simulink model "PIDDiscreto"  (R2021a)
settings: Solver=VariableStepAuto  StartTime=0.0  StopTime=60  RelTol=1e-3
values from neighbouring files (symbols this model uses):
  g = 9.81    [Parcial2PIDDiscreto.m]
  L = 0.25    [Parcial2PIDDiscreto.m]
  m = 0.03    [Parcial2PIDDiscreto.m]
  M = 0.510    (= 0.51)    [Parcial2PIDDiscreto.m]
  ts = 5    [Parcial2PIDDiscreto.m]
  Ts = 0.1    [Parcial2PIDDiscreto.m]
undefined symbols (not defined in the file or in its folder): kdc, kdp, kic, kip, kpc, kpp, Nc, Np
libraries: spsStairGeneratorLib x1
settings Model: Creator=manue  LastModifiedBy=manue

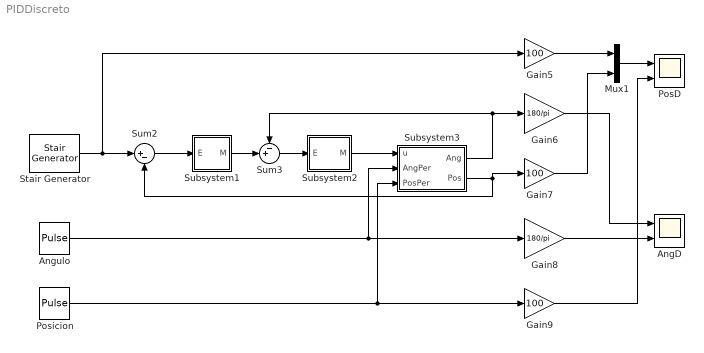
== system PIDDiscreto ==
  AngD : Scope  NumInputPorts=2
  Angulo : DiscretePulseGenerator  PulseType=Time based  Amplitude=10*pi/180  Period=60  PulseWidth=0.1  PhaseDelay=20
  Gain5 : Gain  Gain=100
  Gain6 : Gain  Gain=180/pi
  Gain7 : Gain  Gain=100
  Gain8 : Gain  Gain=180/pi
  Gain9 : Gain  Gain=100
  Mux1 : Mux  Inputs=2
  PosD : Scope  NumInputPorts=2
  Posicion : DiscretePulseGenerator  PulseType=Time based  Amplitude=5/100  Period=60  PhaseDelay=40
  Stair Generator : spsStairGeneratorLib/Stair Generator  t=[0, ts,2*ts,3*ts,4*ts,5*ts,6*ts,7*ts,8*ts,9*ts,10*ts]  e=[25,35,35,40,40,35,35,10,10,30,30]/100  Ts=0
  Subsystem1 : Subsystem
  Subsystem2 : Subsystem
  Subsystem3 : Subsystem
  Sum2 : Sum  Inputs=|+-
  Sum3 : Sum  Inputs=-+|
  wires:
  Gain9/1 -> PosD/2
  Gain5/1 -> Mux1/1
  Posicion/1 -> Subsystem3/3(PosPer), Gain9/1
  Angulo/1 -> Subsystem3/2(AngPer), Gain8/1
  Subsystem3/2(Pos) -> Gain7/1, Sum2/2
  Stair Generator/1 -> Gain5/1, Sum2/1
  Gain6/1 -> AngD/1
  Gain8/1 -> AngD/2
  Subsystem3/1(Ang) -> Sum3/1, Gain6/1
  Gain7/1 -> Mux1/2
  Mux1/1 -> PosD/1
  Sum3/1 -> Subsystem2/1(E)
  Sum2/1 -> Subsystem1/1(E)
  Subsystem1/1(M) -> Sum3/2
  Subsystem2/1(M) -> Subsystem3/1(u)

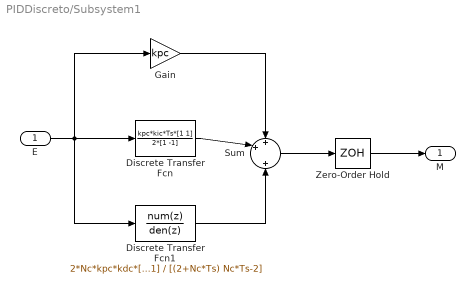
== system PIDDiscreto/Subsystem1 ==
  E : Inport
  Discrete Transfer Fcn : DiscreteTransferFcn  Numerator=kpc*kic*Ts*[1 1]  Denominator=2*[1 -1]  SampleTime=Ts
  Discrete Transfer Fcn1 : DiscreteTransferFcn  Numerator=2*Nc*kpc*kdc*[1 -1]  Denominator=[(2+Nc*Ts) Nc*Ts-2]  SampleTime=Ts
  Gain : Gain  Gain=kpc
  Sum : Sum  Inputs=++|+
  Zero-Order Hold : ZeroOrderHold  SampleTime=Ts
  M : Outport
  wires:
  Discrete Transfer Fcn/1 -> Sum/2
  Discrete Transfer Fcn1/1 -> Sum/3
  Gain/1 -> Sum/1
  Sum/1 -> Zero-Order Hold/1
  Zero-Order Hold/1 -> M/1
  E/1 -> Discrete Transfer Fcn1/1, Discrete Transfer Fcn/1, Gain/1

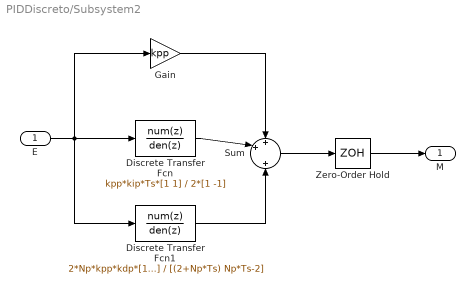
== system PIDDiscreto/Subsystem2 ==
  E : Inport
  Discrete Transfer Fcn : DiscreteTransferFcn  Numerator=kpp*kip*Ts*[1 1]  Denominator=2*[1 -1]  SampleTime=Ts
  Discrete Transfer Fcn1 : DiscreteTransferFcn  Numerator=2*Np*kpp*kdp*[1 -1]  Denominator=[(2+Np*Ts) Np*Ts-2]  SampleTime=Ts
  Gain : Gain  Gain=kpp
  Sum : Sum  Inputs=++|+
  Zero-Order Hold : ZeroOrderHold  SampleTime=Ts
  M : Outport
  wires:
  Zero-Order Hold/1 -> M/1
  Discrete Transfer Fcn1/1 -> Sum/3
  Sum/1 -> Zero-Order Hold/1
  Discrete Transfer Fcn/1 -> Sum/2
  Gain/1 -> Sum/1
  E/1 -> Discrete Transfer Fcn1/1, Discrete Transfer Fcn/1, Gain/1

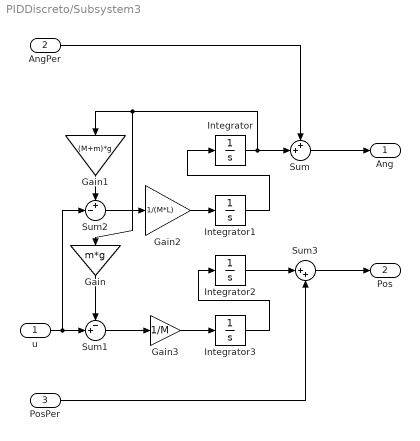
== system PIDDiscreto/Subsystem3 ==
  u : Inport
  AngPer : Inport  Port=2
  PosPer : Inport  Port=3
  Gain : Gain  Gain=m*g
  Gain1 : Gain  Gain=(M+m)*g
  Gain2 : Gain  Gain=1/(M*L)
  Gain3 : Gain  Gain=1/M
  Integrator : Integrator  InitialCondition=10*pi/180
  Integrator1 : Integrator
  Integrator2 : Integrator
  Integrator3 : Integrator
  Sum : Sum  Inputs=++|
  Sum1 : Sum  Inputs=-+|
  Sum2 : Sum  Inputs=+-|
  Sum3 : Sum  Inputs=|++
  Ang : Outport
  Pos : Outport  Port=2
  wires:
  AngPer/1 -> Sum/1
  Integrator/1 -> Gain1/1, Gain/1, Sum/2
  Gain/1 -> Sum1/1
  Gain1/1 -> Sum2/1
  u/1 -> Sum2/2, Sum1/2
  Sum2/1 -> Gain2/1
  Gain2/1 -> Integrator1/1
  Integrator1/1 -> Integrator/1
  Sum1/1 -> Gain3/1
  Gain3/1 -> Integrator3/1
  Integrator3/1 -> Integrator2/1
  Integrator2/1 -> Sum3/1
  PosPer/1 -> Sum3/2
  Sum3/1 -> Pos/1
  Sum/1 -> Ang/1
